simulink model "upCounter"  (R2023b)
settings: Solver=FixedStepAuto  StartTime=0.0  StopTime=Inf  RelTol=1e-3
values from neighbouring files (symbols this model uses):
  maxCnt = 10    [runSLModel.m]    (also in runSLModel_1.m; runSLModel_2.m = 5)
settings Model: SimulationMode=rapid-accelerator  Creator=z004f2se  LastModifiedBy=z004f2se

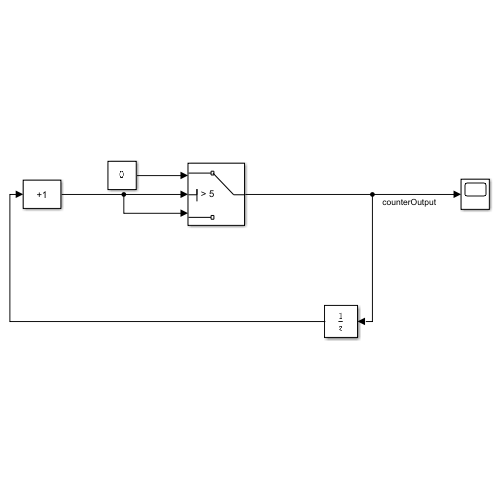
[thumbnail: Simulink's stored preview of the top-level diagram]
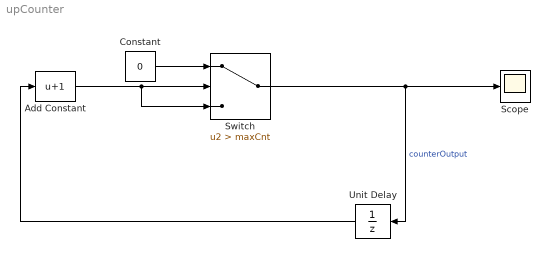
== system upCounter ==
  Add Constant : Bias  Bias=1  SaturateOnIntegerOverflow=off
  Constant : Constant  Value=0
  Scope : Scope
  Switch : Switch  Criteria=u2 > Threshold  Threshold=maxCnt  SaturateOnIntegerOverflow=off  InputSameDT=off
  Unit Delay : UnitDelay  InitialCondition=-1  SampleTime=-1  HasFrameUpgradeWarning=on
  wires:
  Unit Delay/1 -> Add Constant/1
  Switch/1 -> Scope/1, Unit Delay/1  "counterOutput"
  Add Constant/1 -> Switch/3, Switch/2
  Constant/1 -> Switch/1
